simulink model "Team23_project2_week2"  (R2023b)
settings: Solver=VariableStepAuto  StartTime=0.0  StopTime=10.0  RelTol=1e-3
settings Model: Creator=vince  LastModifiedBy=kkern

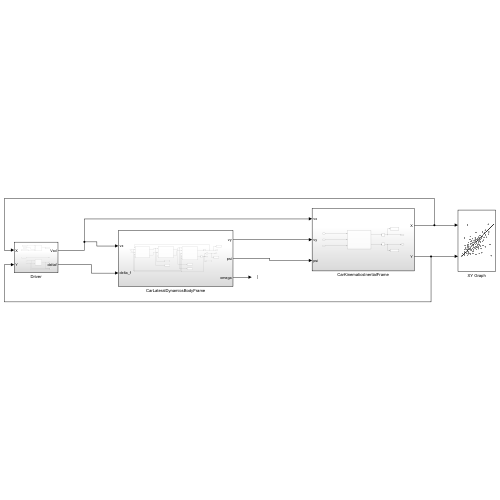
[thumbnail: Simulink's stored preview of the top-level diagram]
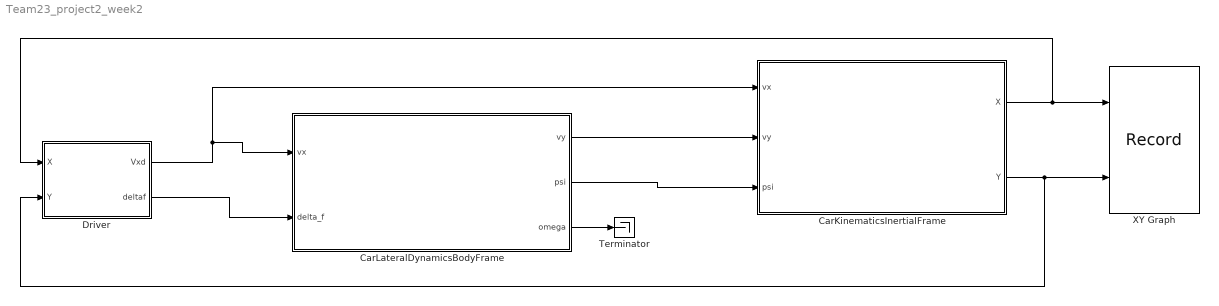
== system Team23_project2_week2 ==
  CarKinematicsInertialFrame : Subsystem
  CarLateralDynamicsBodyFrame : Subsystem
  Driver : Subsystem
  Terminator : Terminator
  XY Graph : Record  FileSettingsInternal="{\"entries\":[{\"content\":{\"excelSettings\":{\"content\":{},\"type\":\"Streamout.ExcelSettings\"}},\"type\":\"Streamout.FileSettingStorage\",\"uuid\":\"\"}],\"packageUris\":[\"http:\\/\\/schema.mathworks.com\\/mf0\\/streamout_blocks\\/R2020a\"],\"version\":\"1.0\"}"  Layout=[1 1]  SignalsInternal="{\"entries\":[{\"content\":{\"signals\":[{\"content\":{\"blockPath\":[],\"dimensions\":[1],\"domain\":\"\",\"lineColor\":\"#a2142f\",\"plots\":[1],\"port\":1,\"signalID\":32,\"signalName\":\"XY Graph:1\"},\"type\":\"RecordBlkView.Signal\",\"uuid\":\"\"},{\"content\":{\"blockPath\":[],\"dimensions\":[1],\"domain\":\"\",\"lineColor\":\"#139fff\",\"plots\":[1],\"port\":2,\"signalID\":35,\"signalName\":\"XY Graph:2\"},\"type\":\"RecordBlkView.Signal\",\"uuid\":\"\"}]},\"type\":\"RecordBlkView.InputSignals\",\"uuid\":\"\"}],\"packageUris\":[\"http:\\/\\/schema.mathworks.com\\/mf0\\/streamout_blocks\\/R2020a\"],\"version\":\"1.0\"}"  VisualizationBindings="{\"xyplotplugin\":{\"info\":[{\"series\":[{\"bindingParametersList\":[{\"parameter\":\"X-Axis\",\"signalID\":32,\"signalName\":\"XY Graph:1\"},{\"parameter\":\"Y-Axis\",\"signalID\":35,\"signalName\":\"XY Graph:2\"}],\"seriesID\":3541}],\"subplotID\":1}]}}"  CompatibilityTag=XY
  wires:
  CarKinematicsInertialFrame/1(X) -> Driver/1(X), XY Graph/1
  CarKinematicsInertialFrame/2(Y) -> Driver/2(Y), XY Graph/2
  CarLateralDynamicsBodyFrame/2(psi) -> CarKinematicsInertialFrame/3(psi)
  CarLateralDynamicsBodyFrame/1(vy) -> CarKinematicsInertialFrame/2(vy)
  Driver/1(Vxd) -> CarKinematicsInertialFrame/1(vx), CarLateralDynamicsBodyFrame/1(vx)
  Driver/2(deltaf) -> CarLateralDynamicsBodyFrame/2(delta_f)
  CarLateralDynamicsBodyFrame/3(omega) -> Terminator/1

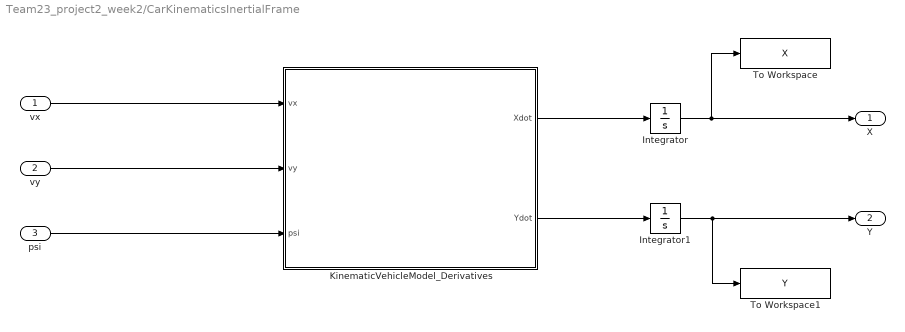
== system Team23_project2_week2/CarKinematicsInertialFrame ==
  vx : Inport
  vy : Inport  Port=2
  psi : Inport  Port=3
  Integrator : Integrator
  Integrator1 : Integrator
  KinematicVehicleModel_Derivatives : MATLAB Function  TreatAsAtomicUnit=on
  To Workspace : ToWorkspace  VariableName=X  SaveFormat=Timeseries  SampleTime=-1
  To Workspace1 : ToWorkspace  VariableName=Y  SaveFormat=Timeseries  SampleTime=-1
  X : Outport
  Y : Outport  Port=2
  wires:
  vx/1 -> KinematicVehicleModel_Derivatives/1(vx)
  vy/1 -> KinematicVehicleModel_Derivatives/2(vy)
  psi/1 -> KinematicVehicleModel_Derivatives/3(psi)
  KinematicVehicleModel_Derivatives/1(Xdot) -> Integrator/1
  KinematicVehicleModel_Derivatives/2(Ydot) -> Integrator1/1
  Integrator/1 -> To Workspace/1, X/1
  Integrator1/1 -> To Workspace1/1, Y/1

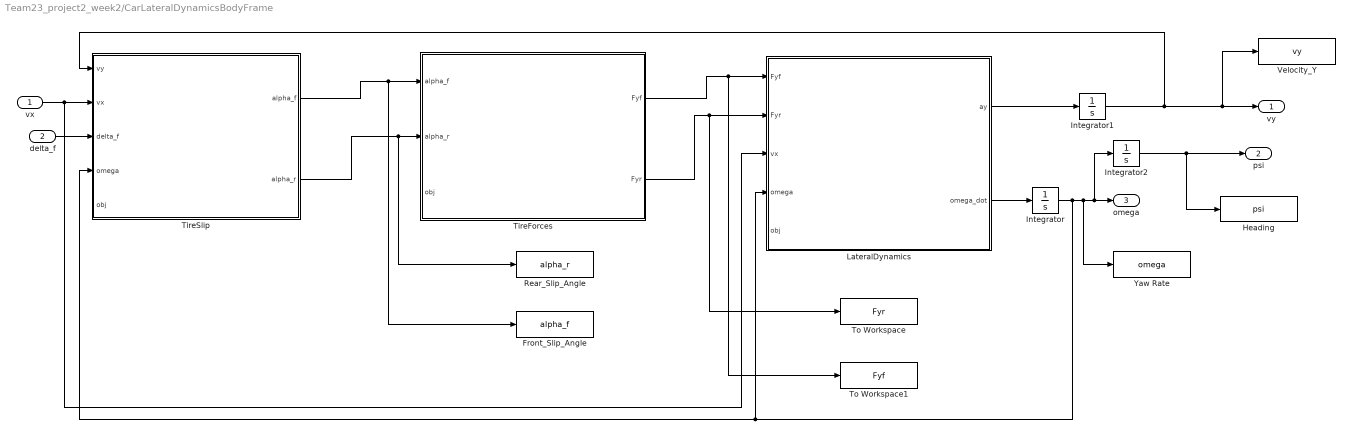
== system Team23_project2_week2/CarLateralDynamicsBodyFrame ==
  vx : Inport
  delta_f : Inport  Port=2
  Front_Slip_Angle : ToWorkspace  VariableName=alpha_f  SaveFormat=Timeseries  SampleTime=-1
  Heading : ToWorkspace  VariableName=psi  SaveFormat=Timeseries  SampleTime=-1
  Integrator : Integrator
  Integrator1 : Integrator
  Integrator2 : Integrator
  LateralDynamics : MATLAB Function  TreatAsAtomicUnit=on
  Rear_Slip_Angle : ToWorkspace  VariableName=alpha_r  SaveFormat=Timeseries  SampleTime=-1
  TireForces : MATLAB Function  TreatAsAtomicUnit=on
  TireSlip : MATLAB Function  TreatAsAtomicUnit=on
  To Workspace : ToWorkspace  VariableName=Fyr  SaveFormat=Timeseries  SampleTime=-1
  To Workspace1 : ToWorkspace  VariableName=Fyf  SaveFormat=Timeseries  SampleTime=-1
  Velocity_Y : ToWorkspace  VariableName=vy  SaveFormat=Timeseries  SampleTime=-1
  Yaw Rate : ToWorkspace  VariableName=omega  SaveFormat=Timeseries  SampleTime=-1
  vy : Outport
  psi : Outport  Port=2
  omega : Outport  Port=3
  wires:
  delta_f/1 -> TireSlip/3(delta_f)
  TireSlip/2(alpha_r) -> Rear_Slip_Angle/1, TireForces/2(alpha_r)
  TireForces/1(Fyf) -> LateralDynamics/1(Fyf), To Workspace1/1
  TireForces/2(Fyr) -> LateralDynamics/2(Fyr), To Workspace/1
  vx/1 -> TireSlip/2(vx), LateralDynamics/3(vx)
  LateralDynamics/1(ay) -> Integrator1/1
  LateralDynamics/2(omega_dot) -> Integrator/1
  Integrator2/1 -> Heading/1, psi/1
  Integrator1/1 -> TireSlip/1(vy), Velocity_Y/1, vy/1
  Integrator/1 -> LateralDynamics/4(omega), TireSlip/4(omega), Yaw Rate/1, Integrator2/1, omega/1
  TireSlip/1(alpha_f) -> TireForces/1(alpha_f), Front_Slip_Angle/1

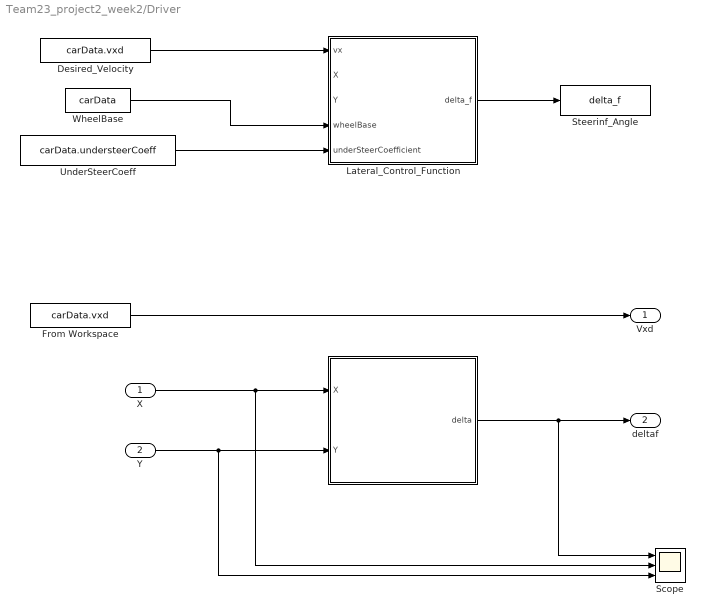
== system Team23_project2_week2/Driver ==
  X : Inport
  Y : Inport  Port=2
  " " : MATLAB Function  TreatAsAtomicUnit=on
  " Lateral_Control_Function" : MATLAB Function  TreatAsAtomicUnit=on
  Desired_Velocity : FromWorkspace  VariableName=carData.vxd
  From Workspace : FromWorkspace  VariableName=carData.vxd
  Scope : Scope  NumInputPorts=3
  Steerinf_Angle : ToWorkspace  VariableName=delta_f  SaveFormat=Timeseries  SampleTime=-1
  UnderSteerCoeff : FromWorkspace  VariableName=carData.understeerCoeff
  WheelBase : FromWorkspace  VariableName=carData
  Vxd : Outport
  deltaf : Outport  Port=2
  wires:
  X/1 -> Scope/2, " "/1(X)
  Y/1 -> Scope/3, " "/2(Y)
  " "/1(delta) -> Scope/1, deltaf/1
  From Workspace/1 -> Vxd/1
  Desired_Velocity/1 -> " Lateral_Control_Function"/1(vx)
  WheelBase/1 -> " Lateral_Control_Function"/4(wheelBase)
  UnderSteerCoeff/1 -> " Lateral_Control_Function"/5(underSteerCoefficient)
  " Lateral_Control_Function"/1(delta_f) -> Steerinf_Angle/1

== matlab function Team23_project2_week2/CarKinematicsInertialFrame/KinematicVehicleModel_Derivatives ==
  data: vx input; Xdot output; vy input; psi input; Ydot output
function [Xdot, Ydot] = fcn(vx, vy, psi)
    temp = TF(psi) * [vx;vy];
    Xdot = temp(1);
    Ydot = temp(2);
end

function y = TF(psi)
    y = [cos(psi), -sin(psi); sin(psi), cos(psi)];
end

== matlab function Team23_project2_week2/Driver/  ==
  data: X input; delta output; Y input
function delta = SimplestDriver(X, Y)

if abs(Y) < 0.5
    delta = 0;
elseif abs(Y - 400) < 0.5
    delta = 0;
elseif X >900
    delta = 5;
else
    delta = -5;
end

== matlab function Team23_project2_week2/CarLateralDynamicsBodyFrame/TireSlip ==
  data: vy input; alpha_f output; vx input; delta_f input; omega input; obj input; alpha_r output
function [alpha_f, alpha_r] = fnc(vy, vx, delta_f, omega, obj)

    if abs(vx) > obj.vx_threshold1
        alpha_f = delta_f - (vy + omega * obj.lf) / vx;
        alpha_r = - (vy - omega * obj.lr) / vx;
    else
        alpha_f = 0;
        alpha_r = 0;
    end

end

== matlab function Team23_project2_week2/CarLateralDynamicsBodyFrame/TireForces ==
  data: alpha_f input; Fyf output; alpha_r input; obj input; Fyr output
function [Fyf, Fyr] = fcn(alpha_f, alpha_r, obj)

    Fyf = min(obj.Fyfmax, obj.Calpha_f * alpha_f);
    Fyr = min(obj.Fyrmax, obj.Calpha_r * alpha_r);

end

== matlab function Team23_project2_week2/CarLateralDynamicsBodyFrame/LateralDynamics ==
  data: Fyf input; ay output; Fyr input; vx input; omega input; obj input; omega_dot output
function [ay, omega_dot] = fcn(Fyf, Fyr, vx, omega, obj)

    Fy = Fyf + Fyr;
    ay = Fy / obj.Mass - omega * vx;

    M = Fyf * obj.lf - Fyr * obj.lr;
    omega_dot = M / obj.Inertia;

end

== matlab function Team23_project2_week2/Driver/ Lateral_Control_Function ==
  data: vx input; X input; delta_f output; Y input; wheelBase input; underSteerCoefficient input
function delta_f = latControl(vx, X, Y, wheelBase, underSteerCoefficient)

track_radius = 200;
track_length = 900;

track_seg1_x0 = 0;
track_seg1_y0 = 0;
track_seg1_x1 = track_length;
track_seg1_y1 = 0;
track_seg2_x0 = track_seg1_x1;
track_seg2_y0 = track_seg1_y1;
track_seg2_x1 = track_seg2_x0;
track_seg2_y1 = track_seg2_y0 + 2 * track_radius;
track_seg3_x0 = track_seg2_x1;
track_seg3_y0 = track_seg2_y1;
track_seg3_x1 = track_seg3_x0 - track_length;
track_seg3_y1 = track_seg3_y0;
track_seg4_x0 = track_seg3_x1;
track_seg4_y0 = track_seg3_y1;
track_seg4_x1 = track_seg1_x0;
track_seg4_y1 = track_seg1_y0;

if X > track_seg1_x0
    if X > track_seg1_x1
        segment = 2;
    else 
        if Y > (track_seg2_y0 + track_seg2_y1)/2
            segment = 3;
        else 
            segment = 1;
        end
    end
else
    segment = 4;
end


switch(segment)
    case 1
        delta_f = 0;
    case 2
        delta_f = - (wheelBase / track_radius + 1 * underSteerCoefficient * vx^2);
    case 3
        delta_f = 0;
    case 4
        delta_f = - (wheelBase / track_radius + 1 * underSteerCoefficient * vx^2);
    otherwise
        delta_f = 0;
end
